simulink model "PlantZoom"  (Simulink 6.1)
settings: Solver=ode45  StartTime=0.0  StopTime=1/testFreq*5  RelTol=1e-3
values from neighbouring files (symbols this model uses):
  delayInquiryZoom = delayImageProc    (= 0.1)    [simZoom.m]
  periodZoomControl = periodFrame * framesPerZoom    (= 0.033)    [simZoom.m]
  pZoom = 1/(1+s/43.3)^4    [simZoom.m]
undefined symbols (not defined in the file or in its folder): zoomRateLimit
settings Model: LastModifiedBy=Big E
settings DebuggingCC: SolverPrmCheckMsg=warning

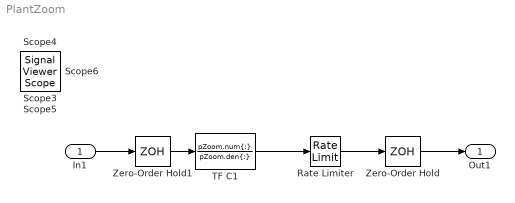
== system PlantZoom ==
  In1 : Inport  Port=1  LatchInput=off
  Rate Limiter : RateLimiter  RisingSlewLimit=zoomRateLimit  FallingSlewLimit=-zoomRateLimit  SampleTimeMode=inherited
  TF C1 : TransferFcn  Numerator=pZoom.num{:}  Denominator=pZoom.den{:}
  Zero-Order Hold : ZeroOrderHold  SampleTime=delayInquiryZoom
  Zero-Order Hold1 : ZeroOrderHold  SampleTime=periodZoomControl
  Out1 : Outport
  Scope{3..6} (4 alike) : SignalViewerScope  IOType=viewer  RefreshTime=0.035000
  wires:
  TF C1/1 -> Rate Limiter/1
  In1/1 -> Zero-Order Hold1/1
  Rate Limiter/1 -> Zero-Order Hold/1
  Zero-Order Hold/1 -> Out1/1
  Zero-Order Hold1/1 -> TF C1/1
